simulink model "pfb_fft"  (Simulink 7.0)
settings: Solver=FixedStepDiscrete  SolverMode=SingleTasking  StartTime=0.0  StopTime=2500  RelTol=1e-3
libraries: xbsIndex_r4 x1144
(part 7 of 20)

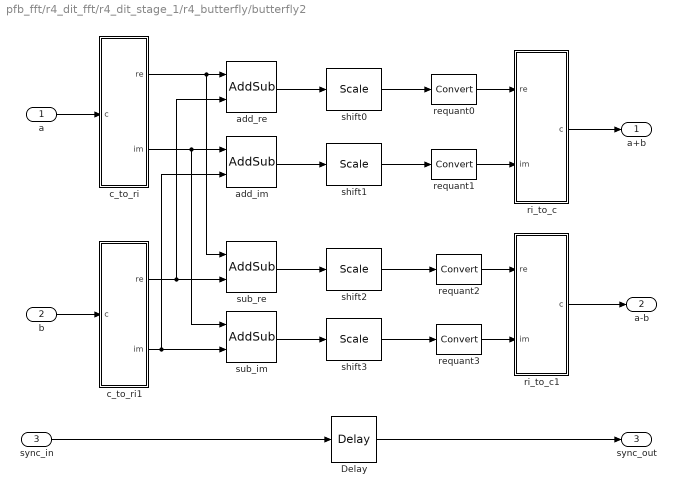
== system pfb_fft/r4_dit_fft/r4_dit_stage_1/r4_butterfly/butterfly2 ==
  a : Inport  OutDataType=sfix(16)  OutScaling=2^0
  b : Inport  Port=2  OutDataType=sfix(16)  OutScaling=2^0
  sync_in : Inport  Port=3  OutDataType=sfix(16)  OutScaling=2^0
  Delay : xbsIndex_r4/Delay  en=off  latency=1  dbl_ovrd=off  reg_retiming=off  block_type=delay
      settings: xl_area=[1 1 0 0 0 0 0]
  add_im : xbsIndex_r4/AddSub  mode=Addition  use_carryin=off  use_carryout=off  en=off  latency=1  precision=Full  arith_type=Unsigned  n_bits=8  bin_pt=2  quantization=Truncate  overflow=Wrap  dbl_ovrd=off  use_behavioral_HDL=on  pipelined=on  use_rpm=on  hw_selection=Fabric  block_type=addsub
      settings: xl_area=[6 11 0 11 0 0 0]  block_version=10.1.3
  add_re : xbsIndex_r4/AddSub  mode=Addition  use_carryin=off  use_carryout=off  en=off  latency=1  precision=Full  arith_type=Unsigned  n_bits=8  bin_pt=2  quantization=Truncate  overflow=Wrap  dbl_ovrd=off  use_behavioral_HDL=on  pipelined=on  use_rpm=on  hw_selection=Fabric  block_type=addsub
      settings: xl_area=[6 11 0 11 0 0 0]  block_version=10.1.3
  c_to_ri : Subsystem  mask(Complex to Real-Imag){n_bits=10, bin_pt=0}
      mask prompts: n_bits "Bit Width"; bin_pt "Binary Point"
      mask help: Outputs real and imaginary components of a complex input.
      settings: AttributesFormatString=10_0 r/i
      mask Help:
      | <pre>
      | Description::
      | 
      | Outputs real and imaginary components of a complex input.
      | Useful for simplifying interconnects.
      | See also: Real-Imag to Complex (ri_to_c)
      | 
      | Mask Parameters::
      | 
      | Bit Width (n_bits): Specifies the width of the real/imaginary components.
      | Assumed equal for both components.
      | 
      | Binary Point (bin_pt): Specifies the binary point location in the real/imaginary components.
      | Assumed equal for both components.
      | </pre>
  c_to_ri1 : Subsystem  mask(Complex to Real-Imag){n_bits=10, bin_pt=0}
      mask prompts: n_bits "Bit Width"; bin_pt "Binary Point"
      mask help: Outputs real and imaginary components of a complex input.
      settings: AttributesFormatString=10_0 r/i
      mask Help:
      | <pre>
      | Description::
      | 
      | Outputs real and imaginary components of a complex input.
      | Useful for simplifying interconnects.
      | See also: Real-Imag to Complex (ri_to_c)
      | 
      | Mask Parameters::
      | 
      | Bit Width (n_bits): Specifies the width of the real/imaginary components.
      | Assumed equal for both components.
      | 
      | Binary Point (bin_pt): Specifies the binary point location in the real/imaginary components.
      | Assumed equal for both components.
      | </pre>
  requant{0..3} (4 alike) : xbsIndex_r4/Convert  arith_type="Signed  (2's comp)"  n_bits=11  bin_pt=0  quantization=Truncate  overflow=Wrap  latency=0  dbl_ovrd=off  pipeline=on  block_type=convert
      settings: xl_area=[0 0 0 0 0 0 0]  block_version=10.1.3
  ri_to_c : Subsystem
      mask Type: Real-Imag to Complex
      mask Description: Concatenates real and imaginary inputs into a complex output.
      mask Help:
      | <pre>
      | Description::
      | 
      | Concatenates a real and imaginary input into a complex output.
      | Useful for simplifying interconnects.
      | See also: Complex to Real-Imag (c_to_ri)
      | 
      | Mask Parameters::
      | 
      | (N/A)
      | </pre>
  ri_to_c1 : Subsystem
      mask Type: Real-Imag to Complex
      mask Description: Concatenates real and imaginary inputs into a complex output.
      mask Help:
      | <pre>
      | Description::
      | 
      | Concatenates a real and imaginary input into a complex output.
      | Useful for simplifying interconnects.
      | See also: Complex to Real-Imag (c_to_ri)
      | 
      | Mask Parameters::
      | 
      | (N/A)
      | </pre>
  shift{0..3} (4 alike) : xbsIndex_r4/Scale  scale_factor=0  dbl_ovrd=off  block_type=scale
      settings: infoedit=Scales input by a power of two by adjusting the binary point position.<P><P>Hardware notes: In hardware this block costs nothing.  block_version=10.1.3
  sub_im : xbsIndex_r4/AddSub  mode=Subtraction  use_carryin=off  use_carryout=off  en=off  latency=1  precision=Full  arith_type=Unsigned  n_bits=8  bin_pt=2  quantization=Truncate  overflow=Wrap  dbl_ovrd=off  use_behavioral_HDL=on  pipelined=on  use_rpm=on  hw_selection=Fabric  block_type=addsub
      settings: xl_area=[6 11 0 11 0 0 0]  block_version=10.1.3
  sub_re : xbsIndex_r4/AddSub  mode=Subtraction  use_carryin=off  use_carryout=off  en=off  latency=1  precision=Full  arith_type=Unsigned  n_bits=8  bin_pt=2  quantization=Truncate  overflow=Wrap  dbl_ovrd=off  use_behavioral_HDL=on  pipelined=on  use_rpm=on  hw_selection=Fabric  block_type=addsub
      settings: xl_area=[6 11 0 11 0 0 0]  block_version=10.1.3
  a+b : Outport  OutDataType=sfix(16)  OutScaling=2^0
  a-b : Outport  Port=2  OutDataType=sfix(16)  OutScaling=2^0
  sync_out : Outport  Port=3  OutDataType=sfix(16)  OutScaling=2^0
  wires:
  shift3/1 -> requant3/1
  sub_im/1 -> shift3/1
  shift2/1 -> requant2/1
  sub_re/1 -> shift2/1
  shift1/1 -> requant1/1
  shift0/1 -> requant0/1
  requant3/1 -> ri_to_c1/2(im)
  requant2/1 -> ri_to_c1/1(re)
  requant1/1 -> ri_to_c/2(im)
  requant0/1 -> ri_to_c/1(re)
  Delay/1 -> sync_out/1
  sync_in/1 -> Delay/1
  ri_to_c1/1(c) -> a-b/1
  ri_to_c/1(c) -> a+b/1
  add_im/1 -> shift1/1
  add_re/1 -> shift0/1
  a/1 -> c_to_ri/1(c)
  c_to_ri/2(im) -> sub_im/1, add_im/1
  c_to_ri/1(re) -> sub_re/1, add_re/1
  c_to_ri1/2(im) -> add_im/2, sub_im/2
  c_to_ri1/1(re) -> add_re/2, sub_re/2
  b/1 -> c_to_ri1/1(c)

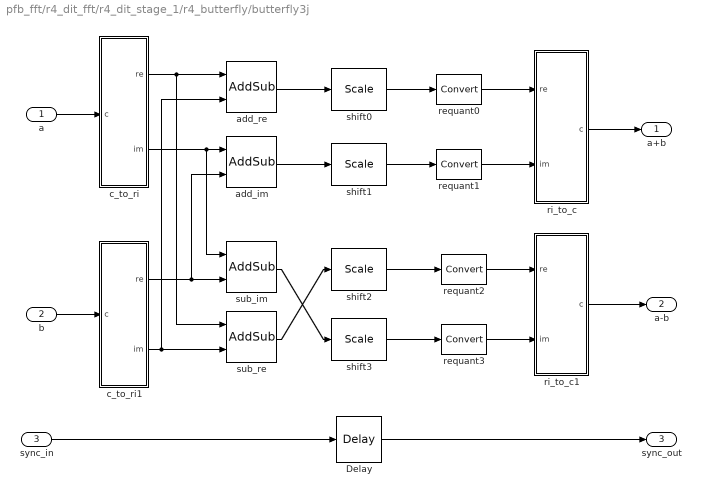
== system pfb_fft/r4_dit_fft/r4_dit_stage_1/r4_butterfly/butterfly3j ==
  a : Inport  OutDataType=sfix(16)  OutScaling=2^0
  b : Inport  Port=2  OutDataType=sfix(16)  OutScaling=2^0
  sync_in : Inport  Port=3  OutDataType=sfix(16)  OutScaling=2^0
  Delay : xbsIndex_r4/Delay  en=off  latency=1  dbl_ovrd=off  reg_retiming=off  block_type=delay
      settings: xl_area=[1 1 0 0 0 0 0]
  add_im : xbsIndex_r4/AddSub  mode=Subtraction  use_carryin=off  use_carryout=off  en=off  latency=1  precision=Full  arith_type=Unsigned  n_bits=8  bin_pt=2  quantization=Truncate  overflow=Wrap  dbl_ovrd=off  use_behavioral_HDL=on  pipelined=on  use_rpm=on  hw_selection=Fabric  block_type=addsub
      settings: xl_area=[6 11 0 11 0 0 0]  block_version=10.1.3
  add_re : xbsIndex_r4/AddSub  mode=Addition  use_carryin=off  use_carryout=off  en=off  latency=1  precision=Full  arith_type=Unsigned  n_bits=8  bin_pt=2  quantization=Truncate  overflow=Wrap  dbl_ovrd=off  use_behavioral_HDL=on  pipelined=on  use_rpm=on  hw_selection=Fabric  block_type=addsub
      settings: xl_area=[6 11 0 11 0 0 0]  block_version=10.1.3
  c_to_ri : Subsystem  mask(Complex to Real-Imag){n_bits=10, bin_pt=0}
      mask prompts: n_bits "Bit Width"; bin_pt "Binary Point"
      mask help: Outputs real and imaginary components of a complex input.
      settings: AttributesFormatString=10_0 r/i
      mask Help:
      | <pre>
      | Description::
      | 
      | Outputs real and imaginary components of a complex input.
      | Useful for simplifying interconnects.
      | See also: Real-Imag to Complex (ri_to_c)
      | 
      | Mask Parameters::
      | 
      | Bit Width (n_bits): Specifies the width of the real/imaginary components.
      | Assumed equal for both components.
      | 
      | Binary Point (bin_pt): Specifies the binary point location in the real/imaginary components.
      | Assumed equal for both components.
      | </pre>
  c_to_ri1 : Subsystem  mask(Complex to Real-Imag){n_bits=10, bin_pt=0}
      mask prompts: n_bits "Bit Width"; bin_pt "Binary Point"
      mask help: Outputs real and imaginary components of a complex input.
      settings: AttributesFormatString=10_0 r/i
      mask Help:
      | <pre>
      | Description::
      | 
      | Outputs real and imaginary components of a complex input.
      | Useful for simplifying interconnects.
      | See also: Real-Imag to Complex (ri_to_c)
      | 
      | Mask Parameters::
      | 
      | Bit Width (n_bits): Specifies the width of the real/imaginary components.
      | Assumed equal for both components.
      | 
      | Binary Point (bin_pt): Specifies the binary point location in the real/imaginary components.
      | Assumed equal for both components.
      | </pre>
  requant{0..3} (4 alike) : xbsIndex_r4/Convert  arith_type="Signed  (2's comp)"  n_bits=11  bin_pt=0  quantization=Truncate  overflow=Wrap  latency=0  dbl_ovrd=off  pipeline=on  block_type=convert
      settings: xl_area=[0 0 0 0 0 0 0]  block_version=10.1.3
  ri_to_c : Subsystem
      mask Type: Real-Imag to Complex
      mask Description: Concatenates real and imaginary inputs into a complex output.
      mask Help:
      | <pre>
      | Description::
      | 
      | Concatenates a real and imaginary input into a complex output.
      | Useful for simplifying interconnects.
      | See also: Complex to Real-Imag (c_to_ri)
      | 
      | Mask Parameters::
      | 
      | (N/A)
      | </pre>
  ri_to_c1 : Subsystem
      mask Type: Real-Imag to Complex
      mask Description: Concatenates real and imaginary inputs into a complex output.
      mask Help:
      | <pre>
      | Description::
      | 
      | Concatenates a real and imaginary input into a complex output.
      | Useful for simplifying interconnects.
      | See also: Complex to Real-Imag (c_to_ri)
      | 
      | Mask Parameters::
      | 
      | (N/A)
      | </pre>
  shift{0..3} (4 alike) : xbsIndex_r4/Scale  scale_factor=0  dbl_ovrd=off  block_type=scale
      settings: infoedit=Scales input by a power of two by adjusting the binary point position.<P><P>Hardware notes: In hardware this block costs nothing.  block_version=10.1.3
  sub_im : xbsIndex_r4/AddSub  mode=Addition  use_carryin=off  use_carryout=off  en=off  latency=1  precision=Full  arith_type=Unsigned  n_bits=8  bin_pt=2  quantization=Truncate  overflow=Wrap  dbl_ovrd=off  use_behavioral_HDL=on  pipelined=on  use_rpm=on  hw_selection=Fabric  block_type=addsub
      settings: xl_area=[6 11 0 11 0 0 0]  block_version=10.1.3
  sub_re : xbsIndex_r4/AddSub  mode=Subtraction  use_carryin=off  use_carryout=off  en=off  latency=1  precision=Full  arith_type=Unsigned  n_bits=8  bin_pt=2  quantization=Truncate  overflow=Wrap  dbl_ovrd=off  use_behavioral_HDL=on  pipelined=on  use_rpm=on  hw_selection=Fabric  block_type=addsub
      settings: xl_area=[6 11 0 11 0 0 0]  block_version=10.1.3
  a+b : Outport  OutDataType=sfix(16)  OutScaling=2^0
  a-b : Outport  Port=2  OutDataType=sfix(16)  OutScaling=2^0
  sync_out : Outport  Port=3  OutDataType=sfix(16)  OutScaling=2^0
  wires:
  requant3/1 -> ri_to_c1/2(im)
  requant2/1 -> ri_to_c1/1(re)
  requant1/1 -> ri_to_c/2(im)
  requant0/1 -> ri_to_c/1(re)
  shift3/1 -> requant3/1
  shift2/1 -> requant2/1
  shift1/1 -> requant1/1
  shift0/1 -> requant0/1
  sub_im/1 -> shift3/1
  sub_re/1 -> shift2/1
  b/1 -> c_to_ri1/1(c)
  c_to_ri1/1(re) -> add_im/2, sub_im/2
  c_to_ri1/2(im) -> add_re/2, sub_re/2
  c_to_ri/1(re) -> sub_re/1, add_re/1
  c_to_ri/2(im) -> sub_im/1, add_im/1
  a/1 -> c_to_ri/1(c)
  add_re/1 -> shift0/1
  add_im/1 -> shift1/1
  ri_to_c/1(c) -> a+b/1
  ri_to_c1/1(c) -> a-b/1
  sync_in/1 -> Delay/1
  Delay/1 -> sync_out/1

== system pfb_fft/r4_dit_fft/r4_dit_stage_2/quadplex_commutator/biplex_commutator_01 ==
  AloAhi : Inport  OutDataType=sfix(16)  OutScaling=2^0
  BloBhi : Inport  Port=2  OutDataType=sfix(16)  OutScaling=2^0
  sync_in : Inport  Port=3  OutDataType=sfix(16)  OutScaling=2^0
  Counter : xbsIndex_r4/Counter  cnt_type=Free Running  cnt_to=Inf  operation=Up  start_count=0  cnt_by_val=1  arith_type=Unsigned  n_bits=7  bin_pt=0  load_pin=off  rst=on  en=off  explicit_period=off  period=1  dbl_ovrd=off  use_behavioral_HDL=off  use_rpm=on  implementation=Fabric  block_type=counter
      settings: xl_area=[4 7 0 7 0 0 0]
  Delay : xbsIndex_r4/Delay  en=off  latency=65  dbl_ovrd=off  reg_retiming=off  block_type=delay
      settings: xl_area=[4 4 0 4 0 0 0]
  Mux : xbsIndex_r4/Mux  inputs=2  en=off  latency=1  precision=Full  arith_type="Signed  (2's comp)"  n_bits=8  bin_pt=2  quantization=Truncate  overflow=Wrap  dbl_ovrd=off  block_type=mux
      settings: xl_area=[11 22 0 22 0 0 0]
  Mux1 : xbsIndex_r4/Mux  inputs=2  en=off  latency=1  precision=Full  arith_type="Signed  (2's comp)"  n_bits=8  bin_pt=2  quantization=Truncate  overflow=Wrap  dbl_ovrd=off  block_type=mux
      settings: xl_area=[11 22 0 22 0 0 0]
  delay_b : Subsystem  mask(Complex Delay){delay_depth=64, n_bits=11, use_bram=on}
      mask prompts: delay_depth "Delay Depth"; n_bits "Bit Width"; use_bram "Use BRAM"
      mask help: A delay block that treats its input as complex, splits it into real and imaginary components, delays each component by a specified amount, and then re-joins them into a complex output. The underlying storage is user-selectable (either BRAM or SLR16 elements).
      settings: AttributesFormatString=|
      | depth = 64
      | delay bram
      mask Help:
      | <pre>
      | Description::
      | 
      | A delay block that treats its input as complex, splits it into real and imaginary components,
      | delays each component by a specified amount, and then re-joins them into a complex
      | output.  The underlying storage is user-selectable (either BRAM or SLR16 elements).
      | 
      | Mask Parameters::
      | 
      | Delay Depth (delay_depth): The length of the delay.
      | 
      | Bit Width (n_bits): Specifies the width of the real/imaginary components.
      | Width of each component is assumed equal.
      | 
      | Use BRAM (use_bram): Check this checkbox to implement the delay using BRAM.
      | If unchecked, the delay will be implemented using SLR16 elements.
      | </pre>
  delay_lo : Subsystem  mask(Complex Delay){delay_depth=64, n_bits=11, use_bram=on}
      mask prompts: delay_depth "Delay Depth"; n_bits "Bit Width"; use_bram "Use BRAM"
      mask help: A delay block that treats its input as complex, splits it into real and imaginary components, delays each component by a specified amount, and then re-joins them into a complex output. The underlying storage is user-selectable (either BRAM or SLR16 elements).
      settings: AttributesFormatString=|
      | depth = 64
      | delay bram
      mask Help:
      | <pre>
      | Description::
      | 
      | A delay block that treats its input as complex, splits it into real and imaginary components,
      | delays each component by a specified amount, and then re-joins them into a complex
      | output.  The underlying storage is user-selectable (either BRAM or SLR16 elements).
      | 
      | Mask Parameters::
      | 
      | Delay Depth (delay_depth): The length of the delay.
      | 
      | Bit Width (n_bits): Specifies the width of the real/imaginary components.
      | Width of each component is assumed equal.
      | 
      | Use BRAM (use_bram): Check this checkbox to implement the delay using BRAM.
      | If unchecked, the delay will be implemented using SLR16 elements.
      | </pre>
  top_bit : xbsIndex_r4/Slice  nbits=1  boolean_output=off  mode=Upper Bit Location + Width  bit1=0  base1=MSB of Input  bit0=0  base0=LSB of Input  dbl_ovrd=off  block_type=slice
      settings: infoedit="Extracts a given range of bits from each input sample and presents it at the output.  The output type is ordinarily unsigned with binary point at zero, but can be Boolean when the slice is one bit wide.<P><P>Hardware notes: In hardware this block costs nothing."  block_version=10.1.3
  AloBlo : Outport  OutDataType=sfix(16)  OutScaling=2^0
  AhiBhi : Outport  Port=2  OutDataType=sfix(16)  OutScaling=2^0
  sync_out : Outport  Port=3  OutDataType=sfix(16)  OutScaling=2^0
  wires:
  Delay/1 -> sync_out/1
  delay_lo/1(out) -> AloBlo/1
  Mux/1 -> delay_lo/1(in)
  delay_b/1(out) -> Mux/3, Mux1/2
  BloBhi/1 -> delay_b/1(in)
  Mux1/1 -> AhiBhi/1
  AloAhi/1 -> Mux1/3, Mux/2
  top_bit/1 -> Mux/1, Mux1/1
  Counter/1 -> top_bit/1
  sync_in/1 -> Delay/1, Counter/1

== system pfb_fft/r4_dit_fft/r4_dit_stage_2/quadplex_commutator/biplex_commutator_23 ==
  AloAhi : Inport  OutDataType=sfix(16)  OutScaling=2^0
  BloBhi : Inport  Port=2  OutDataType=sfix(16)  OutScaling=2^0
  sync_in : Inport  Port=3  OutDataType=sfix(16)  OutScaling=2^0
  Counter : xbsIndex_r4/Counter  cnt_type=Free Running  cnt_to=Inf  operation=Up  start_count=0  cnt_by_val=1  arith_type=Unsigned  n_bits=7  bin_pt=0  load_pin=off  rst=on  en=off  explicit_period=off  period=1  dbl_ovrd=off  use_behavioral_HDL=off  use_rpm=on  implementation=Fabric  block_type=counter
      settings: xl_area=[4 7 0 7 0 0 0]
  Delay : xbsIndex_r4/Delay  en=off  latency=65  dbl_ovrd=off  reg_retiming=off  block_type=delay
      settings: xl_area=[4 4 0 4 0 0 0]
  Mux : xbsIndex_r4/Mux  inputs=2  en=off  latency=1  precision=Full  arith_type="Signed  (2's comp)"  n_bits=8  bin_pt=2  quantization=Truncate  overflow=Wrap  dbl_ovrd=off  block_type=mux
      settings: xl_area=[11 22 0 22 0 0 0]
  Mux1 : xbsIndex_r4/Mux  inputs=2  en=off  latency=1  precision=Full  arith_type="Signed  (2's comp)"  n_bits=8  bin_pt=2  quantization=Truncate  overflow=Wrap  dbl_ovrd=off  block_type=mux
      settings: xl_area=[11 22 0 22 0 0 0]
  delay_b : Subsystem  mask(Complex Delay){delay_depth=64, n_bits=11, use_bram=on}
      mask prompts: delay_depth "Delay Depth"; n_bits "Bit Width"; use_bram "Use BRAM"
      mask help: A delay block that treats its input as complex, splits it into real and imaginary components, delays each component by a specified amount, and then re-joins them into a complex output. The underlying storage is user-selectable (either BRAM or SLR16 elements).
      settings: AttributesFormatString=|
      | depth = 64
      | delay bram
      mask Help:
      | <pre>
      | Description::
      | 
      | A delay block that treats its input as complex, splits it into real and imaginary components,
      | delays each component by a specified amount, and then re-joins them into a complex
      | output.  The underlying storage is user-selectable (either BRAM or SLR16 elements).
      | 
      | Mask Parameters::
      | 
      | Delay Depth (delay_depth): The length of the delay.
      | 
      | Bit Width (n_bits): Specifies the width of the real/imaginary components.
      | Width of each component is assumed equal.
      | 
      | Use BRAM (use_bram): Check this checkbox to implement the delay using BRAM.
      | If unchecked, the delay will be implemented using SLR16 elements.
      | </pre>
  delay_lo : Subsystem  mask(Complex Delay){delay_depth=64, n_bits=11, use_bram=on}
      mask prompts: delay_depth "Delay Depth"; n_bits "Bit Width"; use_bram "Use BRAM"
      mask help: A delay block that treats its input as complex, splits it into real and imaginary components, delays each component by a specified amount, and then re-joins them into a complex output. The underlying storage is user-selectable (either BRAM or SLR16 elements).
      settings: AttributesFormatString=|
      | depth = 64
      | delay bram
      mask Help:
      | <pre>
      | Description::
      | 
      | A delay block that treats its input as complex, splits it into real and imaginary components,
      | delays each component by a specified amount, and then re-joins them into a complex
      | output.  The underlying storage is user-selectable (either BRAM or SLR16 elements).
      | 
      | Mask Parameters::
      | 
      | Delay Depth (delay_depth): The length of the delay.
      | 
      | Bit Width (n_bits): Specifies the width of the real/imaginary components.
      | Width of each component is assumed equal.
      | 
      | Use BRAM (use_bram): Check this checkbox to implement the delay using BRAM.
      | If unchecked, the delay will be implemented using SLR16 elements.
      | </pre>
  top_bit : xbsIndex_r4/Slice  nbits=1  boolean_output=off  mode=Upper Bit Location + Width  bit1=0  base1=MSB of Input  bit0=0  base0=LSB of Input  dbl_ovrd=off  block_type=slice
      settings: infoedit="Extracts a given range of bits from each input sample and presents it at the output.  The output type is ordinarily unsigned with binary point at zero, but can be Boolean when the slice is one bit wide.<P><P>Hardware notes: In hardware this block costs nothing."  block_version=10.1.3
  AloBlo : Outport  OutDataType=sfix(16)  OutScaling=2^0
  AhiBhi : Outport  Port=2  OutDataType=sfix(16)  OutScaling=2^0
  sync_out : Outport  Port=3  OutDataType=sfix(16)  OutScaling=2^0
  wires:
  Delay/1 -> sync_out/1
  delay_lo/1(out) -> AloBlo/1
  Mux/1 -> delay_lo/1(in)
  delay_b/1(out) -> Mux/3, Mux1/2
  BloBhi/1 -> delay_b/1(in)
  Mux1/1 -> AhiBhi/1
  AloAhi/1 -> Mux1/3, Mux/2
  top_bit/1 -> Mux/1, Mux1/1
  Counter/1 -> top_bit/1
  sync_in/1 -> Delay/1, Counter/1

== system pfb_fft/r4_dit_fft/r4_dit_stage_2/quadplex_commutator/biplex_commutator_ac ==
  AloAhi : Inport  OutDataType=sfix(16)  OutScaling=2^0
  BloBhi : Inport  Port=2  OutDataType=sfix(16)  OutScaling=2^0
  sync_in : Inport  Port=3  OutDataType=sfix(16)  OutScaling=2^0
  Counter : xbsIndex_r4/Counter  cnt_type=Free Running  cnt_to=Inf  operation=Up  start_count=0  cnt_by_val=1  arith_type=Unsigned  n_bits=8  bin_pt=0  load_pin=off  rst=on  en=off  explicit_period=off  period=1  dbl_ovrd=off  use_behavioral_HDL=off  use_rpm=on  implementation=Fabric  block_type=counter
      settings: xl_area=[4 8 0 8 0 0 0]
  Delay : xbsIndex_r4/Delay  en=off  latency=129  dbl_ovrd=off  reg_retiming=off  block_type=delay
      settings: xl_area=[8 8 0 8 0 0 0]
  Mux : xbsIndex_r4/Mux  inputs=2  en=off  latency=1  precision=Full  arith_type="Signed  (2's comp)"  n_bits=8  bin_pt=2  quantization=Truncate  overflow=Wrap  dbl_ovrd=off  block_type=mux
      settings: xl_area=[11 22 0 22 0 0 0]
  Mux1 : xbsIndex_r4/Mux  inputs=2  en=off  latency=1  precision=Full  arith_type="Signed  (2's comp)"  n_bits=8  bin_pt=2  quantization=Truncate  overflow=Wrap  dbl_ovrd=off  block_type=mux
      settings: xl_area=[11 22 0 22 0 0 0]
  delay_b : Subsystem  mask(Complex Delay){delay_depth=128, n_bits=11, use_bram=on}
      mask prompts: delay_depth "Delay Depth"; n_bits "Bit Width"; use_bram "Use BRAM"
      mask help: A delay block that treats its input as complex, splits it into real and imaginary components, delays each component by a specified amount, and then re-joins them into a complex output. The underlying storage is user-selectable (either BRAM or SLR16 elements).
      settings: AttributesFormatString=|
      | depth = 128
      | delay bram
      mask Help:
      | <pre>
      | Description::
      | 
      | A delay block that treats its input as complex, splits it into real and imaginary components,
      | delays each component by a specified amount, and then re-joins them into a complex
      | output.  The underlying storage is user-selectable (either BRAM or SLR16 elements).
      | 
      | Mask Parameters::
      | 
      | Delay Depth (delay_depth): The length of the delay.
      | 
      | Bit Width (n_bits): Specifies the width of the real/imaginary components.
      | Width of each component is assumed equal.
      | 
      | Use BRAM (use_bram): Check this checkbox to implement the delay using BRAM.
      | If unchecked, the delay will be implemented using SLR16 elements.
      | </pre>
  delay_lo : Subsystem  mask(Complex Delay){delay_depth=128, n_bits=11, use_bram=on}
      mask prompts: delay_depth "Delay Depth"; n_bits "Bit Width"; use_bram "Use BRAM"
      mask help: A delay block that treats its input as complex, splits it into real and imaginary components, delays each component by a specified amount, and then re-joins them into a complex output. The underlying storage is user-selectable (either BRAM or SLR16 elements).
      settings: AttributesFormatString=|
      | depth = 128
      | delay bram
      mask Help:
      | <pre>
      | Description::
      | 
      | A delay block that treats its input as complex, splits it into real and imaginary components,
      | delays each component by a specified amount, and then re-joins them into a complex
      | output.  The underlying storage is user-selectable (either BRAM or SLR16 elements).
      | 
      | Mask Parameters::
      | 
      | Delay Depth (delay_depth): The length of the delay.
      | 
      | Bit Width (n_bits): Specifies the width of the real/imaginary components.
      | Width of each component is assumed equal.
      | 
      | Use BRAM (use_bram): Check this checkbox to implement the delay using BRAM.
      | If unchecked, the delay will be implemented using SLR16 elements.
      | </pre>
  top_bit : xbsIndex_r4/Slice  nbits=1  boolean_output=off  mode=Upper Bit Location + Width  bit1=0  base1=MSB of Input  bit0=0  base0=LSB of Input  dbl_ovrd=off  block_type=slice
      settings: infoedit="Extracts a given range of bits from each input sample and presents it at the output.  The output type is ordinarily unsigned with binary point at zero, but can be Boolean when the slice is one bit wide.<P><P>Hardware notes: In hardware this block costs nothing."  block_version=10.1.3
  AloBlo : Outport  OutDataType=sfix(16)  OutScaling=2^0
  AhiBhi : Outport  Port=2  OutDataType=sfix(16)  OutScaling=2^0
  sync_out : Outport  Port=3  OutDataType=sfix(16)  OutScaling=2^0
  wires:
  Delay/1 -> sync_out/1
  delay_lo/1(out) -> AloBlo/1
  Mux/1 -> delay_lo/1(in)
  delay_b/1(out) -> Mux/3, Mux1/2
  BloBhi/1 -> delay_b/1(in)
  Mux1/1 -> AhiBhi/1
  AloAhi/1 -> Mux1/3, Mux/2
  top_bit/1 -> Mux/1, Mux1/1
  Counter/1 -> top_bit/1
  sync_in/1 -> Delay/1, Counter/1

== system pfb_fft/r4_dit_fft/r4_dit_stage_2/quadplex_commutator/biplex_commutator_bd ==
  AloAhi : Inport  OutDataType=sfix(16)  OutScaling=2^0
  BloBhi : Inport  Port=2  OutDataType=sfix(16)  OutScaling=2^0
  sync_in : Inport  Port=3  OutDataType=sfix(16)  OutScaling=2^0
  Counter : xbsIndex_r4/Counter  cnt_type=Free Running  cnt_to=Inf  operation=Up  start_count=0  cnt_by_val=1  arith_type=Unsigned  n_bits=8  bin_pt=0  load_pin=off  rst=on  en=off  explicit_period=off  period=1  dbl_ovrd=off  use_behavioral_HDL=off  use_rpm=on  implementation=Fabric  block_type=counter
      settings: xl_area=[4 8 0 8 0 0 0]
  Delay : xbsIndex_r4/Delay  en=off  latency=129  dbl_ovrd=off  reg_retiming=off  block_type=delay
      settings: xl_area=[8 8 0 8 0 0 0]
  Mux : xbsIndex_r4/Mux  inputs=2  en=off  latency=1  precision=Full  arith_type="Signed  (2's comp)"  n_bits=8  bin_pt=2  quantization=Truncate  overflow=Wrap  dbl_ovrd=off  block_type=mux
      settings: xl_area=[11 22 0 22 0 0 0]
  Mux1 : xbsIndex_r4/Mux  inputs=2  en=off  latency=1  precision=Full  arith_type="Signed  (2's comp)"  n_bits=8  bin_pt=2  quantization=Truncate  overflow=Wrap  dbl_ovrd=off  block_type=mux
      settings: xl_area=[11 22 0 22 0 0 0]
  delay_b : Subsystem  mask(Complex Delay){delay_depth=128, n_bits=11, use_bram=on}
      mask prompts: delay_depth "Delay Depth"; n_bits "Bit Width"; use_bram "Use BRAM"
      mask help: A delay block that treats its input as complex, splits it into real and imaginary components, delays each component by a specified amount, and then re-joins them into a complex output. The underlying storage is user-selectable (either BRAM or SLR16 elements).
      settings: AttributesFormatString=|
      | depth = 128
      | delay bram
      mask Help:
      | <pre>
      | Description::
      | 
      | A delay block that treats its input as complex, splits it into real and imaginary components,
      | delays each component by a specified amount, and then re-joins them into a complex
      | output.  The underlying storage is user-selectable (either BRAM or SLR16 elements).
      | 
      | Mask Parameters::
      | 
      | Delay Depth (delay_depth): The length of the delay.
      | 
      | Bit Width (n_bits): Specifies the width of the real/imaginary components.
      | Width of each component is assumed equal.
      | 
      | Use BRAM (use_bram): Check this checkbox to implement the delay using BRAM.
      | If unchecked, the delay will be implemented using SLR16 elements.
      | </pre>
  delay_lo : Subsystem  mask(Complex Delay){delay_depth=128, n_bits=11, use_bram=on}
      mask prompts: delay_depth "Delay Depth"; n_bits "Bit Width"; use_bram "Use BRAM"
      mask help: A delay block that treats its input as complex, splits it into real and imaginary components, delays each component by a specified amount, and then re-joins them into a complex output. The underlying storage is user-selectable (either BRAM or SLR16 elements).
      settings: AttributesFormatString=|
      | depth = 128
      | delay bram
      mask Help:
      | <pre>
      | Description::
      | 
      | A delay block that treats its input as complex, splits it into real and imaginary components,
      | delays each component by a specified amount, and then re-joins them into a complex
      | output.  The underlying storage is user-selectable (either BRAM or SLR16 elements).
      | 
      | Mask Parameters::
      | 
      | Delay Depth (delay_depth): The length of the delay.
      | 
      | Bit Width (n_bits): Specifies the width of the real/imaginary components.
      | Width of each component is assumed equal.
      | 
      | Use BRAM (use_bram): Check this checkbox to implement the delay using BRAM.
      | If unchecked, the delay will be implemented using SLR16 elements.
      | </pre>
  top_bit : xbsIndex_r4/Slice  nbits=1  boolean_output=off  mode=Upper Bit Location + Width  bit1=0  base1=MSB of Input  bit0=0  base0=LSB of Input  dbl_ovrd=off  block_type=slice
      settings: infoedit="Extracts a given range of bits from each input sample and presents it at the output.  The output type is ordinarily unsigned with binary point at zero, but can be Boolean when the slice is one bit wide.<P><P>Hardware notes: In hardware this block costs nothing."  block_version=10.1.3
  AloBlo : Outport  OutDataType=sfix(16)  OutScaling=2^0
  AhiBhi : Outport  Port=2  OutDataType=sfix(16)  OutScaling=2^0
  sync_out : Outport  Port=3  OutDataType=sfix(16)  OutScaling=2^0
  wires:
  Delay/1 -> sync_out/1
  delay_lo/1(out) -> AloBlo/1
  Mux/1 -> delay_lo/1(in)
  delay_b/1(out) -> Mux/3, Mux1/2
  BloBhi/1 -> delay_b/1(in)
  Mux1/1 -> AhiBhi/1
  AloAhi/1 -> Mux1/3, Mux/2
  top_bit/1 -> Mux/1, Mux1/1
  Counter/1 -> top_bit/1
  sync_in/1 -> Delay/1, Counter/1

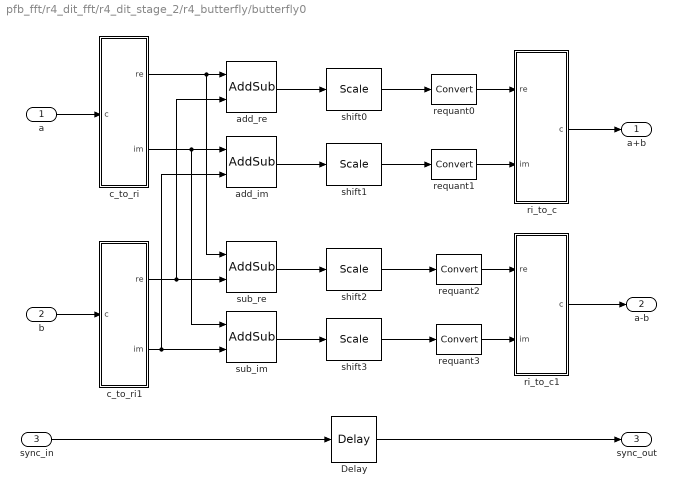
== system pfb_fft/r4_dit_fft/r4_dit_stage_2/r4_butterfly/butterfly0 ==
  a : Inport  OutDataType=sfix(16)  OutScaling=2^0
  b : Inport  Port=2  OutDataType=sfix(16)  OutScaling=2^0
  sync_in : Inport  Port=3  OutDataType=sfix(16)  OutScaling=2^0
  Delay : xbsIndex_r4/Delay  en=off  latency=1  dbl_ovrd=off  reg_retiming=off  block_type=delay
      settings: xl_area=[1 1 0 0 0 0 0]
  add_im : xbsIndex_r4/AddSub  mode=Addition  use_carryin=off  use_carryout=off  en=off  latency=1  precision=Full  arith_type=Unsigned  n_bits=8  bin_pt=2  quantization=Truncate  overflow=Wrap  dbl_ovrd=off  use_behavioral_HDL=on  pipelined=on  use_rpm=on  hw_selection=Fabric  block_type=addsub
      settings: xl_area=[6 12 0 12 0 0 0]  block_version=10.1.3
  add_re : xbsIndex_r4/AddSub  mode=Addition  use_carryin=off  use_carryout=off  en=off  latency=1  precision=Full  arith_type=Unsigned  n_bits=8  bin_pt=2  quantization=Truncate  overflow=Wrap  dbl_ovrd=off  use_behavioral_HDL=on  pipelined=on  use_rpm=on  hw_selection=Fabric  block_type=addsub
      settings: xl_area=[6 12 0 12 0 0 0]  block_version=10.1.3
  c_to_ri : Subsystem  mask(Complex to Real-Imag){n_bits=11, bin_pt=0}
      mask prompts: n_bits "Bit Width"; bin_pt "Binary Point"
      mask help: Outputs real and imaginary components of a complex input.
      settings: AttributesFormatString=11_0 r/i
      mask Help:
      | <pre>
      | Description::
      | 
      | Outputs real and imaginary components of a complex input.
      | Useful for simplifying interconnects.
      | See also: Real-Imag to Complex (ri_to_c)
      | 
      | Mask Parameters::
      | 
      | Bit Width (n_bits): Specifies the width of the real/imaginary components.
      | Assumed equal for both components.
      | 
      | Binary Point (bin_pt): Specifies the binary point location in the real/imaginary components.
      | Assumed equal for both components.
      | </pre>
  c_to_ri1 : Subsystem  mask(Complex to Real-Imag){n_bits=11, bin_pt=0}
      mask prompts: n_bits "Bit Width"; bin_pt "Binary Point"
      mask help: Outputs real and imaginary components of a complex input.
      settings: AttributesFormatString=11_0 r/i
      mask Help:
      | <pre>
      | Description::
      | 
      | Outputs real and imaginary components of a complex input.
      | Useful for simplifying interconnects.
      | See also: Real-Imag to Complex (ri_to_c)
      | 
      | Mask Parameters::
      | 
      | Bit Width (n_bits): Specifies the width of the real/imaginary components.
      | Assumed equal for both components.
      | 
      | Binary Point (bin_pt): Specifies the binary point location in the real/imaginary components.
      | Assumed equal for both components.
      | </pre>
  requant{0..3} (4 alike) : xbsIndex_r4/Convert  arith_type="Signed  (2's comp)"  n_bits=12  bin_pt=0  quantization=Truncate  overflow=Wrap  latency=0  dbl_ovrd=off  pipeline=on  block_type=convert
      settings: xl_area=[0 0 0 0 0 0 0]  block_version=10.1.3
  ri_to_c : Subsystem
      mask Type: Real-Imag to Complex
      mask Description: Concatenates real and imaginary inputs into a complex output.
      mask Help:
      | <pre>
      | Description::
      | 
      | Concatenates a real and imaginary input into a complex output.
      | Useful for simplifying interconnects.
      | See also: Complex to Real-Imag (c_to_ri)
      | 
      | Mask Parameters::
      | 
      | (N/A)
      | </pre>
  ri_to_c1 : Subsystem
      mask Type: Real-Imag to Complex
      mask Description: Concatenates real and imaginary inputs into a complex output.
      mask Help:
      | <pre>
      | Description::
      | 
      | Concatenates a real and imaginary input into a complex output.
      | Useful for simplifying interconnects.
      | See also: Complex to Real-Imag (c_to_ri)
      | 
      | Mask Parameters::
      | 
      | (N/A)
      | </pre>
  shift{0..3} (4 alike) : xbsIndex_r4/Scale  scale_factor=0  dbl_ovrd=off  block_type=scale
      settings: infoedit=Scales input by a power of two by adjusting the binary point position.<P><P>Hardware notes: In hardware this block costs nothing.  block_version=10.1.3
  sub_im : xbsIndex_r4/AddSub  mode=Subtraction  use_carryin=off  use_carryout=off  en=off  latency=1  precision=Full  arith_type=Unsigned  n_bits=8  bin_pt=2  quantization=Truncate  overflow=Wrap  dbl_ovrd=off  use_behavioral_HDL=on  pipelined=on  use_rpm=on  hw_selection=Fabric  block_type=addsub
      settings: xl_area=[6 12 0 12 0 0 0]  block_version=10.1.3
  sub_re : xbsIndex_r4/AddSub  mode=Subtraction  use_carryin=off  use_carryout=off  en=off  latency=1  precision=Full  arith_type=Unsigned  n_bits=8  bin_pt=2  quantization=Truncate  overflow=Wrap  dbl_ovrd=off  use_behavioral_HDL=on  pipelined=on  use_rpm=on  hw_selection=Fabric  block_type=addsub
      settings: xl_area=[6 12 0 12 0 0 0]  block_version=10.1.3
  a+b : Outport  OutDataType=sfix(16)  OutScaling=2^0
  a-b : Outport  Port=2  OutDataType=sfix(16)  OutScaling=2^0
  sync_out : Outport  Port=3  OutDataType=sfix(16)  OutScaling=2^0
  wires:
  shift3/1 -> requant3/1
  sub_im/1 -> shift3/1
  shift2/1 -> requant2/1
  sub_re/1 -> shift2/1
  shift1/1 -> requant1/1
  shift0/1 -> requant0/1
  requant3/1 -> ri_to_c1/2(im)
  requant2/1 -> ri_to_c1/1(re)
  requant1/1 -> ri_to_c/2(im)
  requant0/1 -> ri_to_c/1(re)
  Delay/1 -> sync_out/1
  sync_in/1 -> Delay/1
  ri_to_c1/1(c) -> a-b/1
  ri_to_c/1(c) -> a+b/1
  add_im/1 -> shift1/1
  add_re/1 -> shift0/1
  a/1 -> c_to_ri/1(c)
  c_to_ri/2(im) -> sub_im/1, add_im/1
  c_to_ri/1(re) -> sub_re/1, add_re/1
  c_to_ri1/2(im) -> add_im/2, sub_im/2
  c_to_ri1/1(re) -> add_re/2, sub_re/2
  b/1 -> c_to_ri1/1(c)

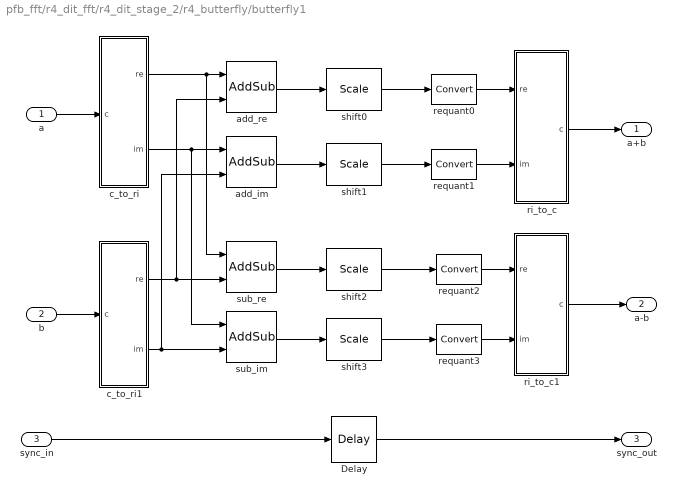
== system pfb_fft/r4_dit_fft/r4_dit_stage_2/r4_butterfly/butterfly1 ==
  a : Inport  OutDataType=sfix(16)  OutScaling=2^0
  b : Inport  Port=2  OutDataType=sfix(16)  OutScaling=2^0
  sync_in : Inport  Port=3  OutDataType=sfix(16)  OutScaling=2^0
  Delay : xbsIndex_r4/Delay  en=off  latency=1  dbl_ovrd=off  reg_retiming=off  block_type=delay
      settings: xl_area=[1 1 0 0 0 0 0]
  add_im : xbsIndex_r4/AddSub  mode=Addition  use_carryin=off  use_carryout=off  en=off  latency=1  precision=Full  arith_type=Unsigned  n_bits=8  bin_pt=2  quantization=Truncate  overflow=Wrap  dbl_ovrd=off  use_behavioral_HDL=on  pipelined=on  use_rpm=on  hw_selection=Fabric  block_type=addsub
      settings: xl_area=[6 12 0 12 0 0 0]  block_version=10.1.3
  add_re : xbsIndex_r4/AddSub  mode=Addition  use_carryin=off  use_carryout=off  en=off  latency=1  precision=Full  arith_type=Unsigned  n_bits=8  bin_pt=2  quantization=Truncate  overflow=Wrap  dbl_ovrd=off  use_behavioral_HDL=on  pipelined=on  use_rpm=on  hw_selection=Fabric  block_type=addsub
      settings: xl_area=[6 12 0 12 0 0 0]  block_version=10.1.3
  c_to_ri : Subsystem  mask(Complex to Real-Imag){n_bits=11, bin_pt=0}
      mask prompts: n_bits "Bit Width"; bin_pt "Binary Point"
      mask help: Outputs real and imaginary components of a complex input.
      settings: AttributesFormatString=11_0 r/i
      mask Help:
      | <pre>
      | Description::
      | 
      | Outputs real and imaginary components of a complex input.
      | Useful for simplifying interconnects.
      | See also: Real-Imag to Complex (ri_to_c)
      | 
      | Mask Parameters::
      | 
      | Bit Width (n_bits): Specifies the width of the real/imaginary components.
      | Assumed equal for both components.
      | 
      | Binary Point (bin_pt): Specifies the binary point location in the real/imaginary components.
      | Assumed equal for both components.
      | </pre>
  c_to_ri1 : Subsystem  mask(Complex to Real-Imag){n_bits=11, bin_pt=0}
      mask prompts: n_bits "Bit Width"; bin_pt "Binary Point"
      mask help: Outputs real and imaginary components of a complex input.
      settings: AttributesFormatString=11_0 r/i
      mask Help:
      | <pre>
      | Description::
      | 
      | Outputs real and imaginary components of a complex input.
      | Useful for simplifying interconnects.
      | See also: Real-Imag to Complex (ri_to_c)
      | 
      | Mask Parameters::
      | 
      | Bit Width (n_bits): Specifies the width of the real/imaginary components.
      | Assumed equal for both components.
      | 
      | Binary Point (bin_pt): Specifies the binary point location in the real/imaginary components.
      | Assumed equal for both components.
      | </pre>
  requant{0..3} (4 alike) : xbsIndex_r4/Convert  arith_type="Signed  (2's comp)"  n_bits=12  bin_pt=0  quantization=Truncate  overflow=Wrap  latency=0  dbl_ovrd=off  pipeline=on  block_type=convert
      settings: xl_area=[0 0 0 0 0 0 0]  block_version=10.1.3
  ri_to_c : Subsystem
      mask Type: Real-Imag to Complex
      mask Description: Concatenates real and imaginary inputs into a complex output.
      mask Help:
      | <pre>
      | Description::
      | 
      | Concatenates a real and imaginary input into a complex output.
      | Useful for simplifying interconnects.
      | See also: Complex to Real-Imag (c_to_ri)
      | 
      | Mask Parameters::
      | 
      | (N/A)
      | </pre>
  ri_to_c1 : Subsystem
      mask Type: Real-Imag to Complex
      mask Description: Concatenates real and imaginary inputs into a complex output.
      mask Help:
      | <pre>
      | Description::
      | 
      | Concatenates a real and imaginary input into a complex output.
      | Useful for simplifying interconnects.
      | See also: Complex to Real-Imag (c_to_ri)
      | 
      | Mask Parameters::
      | 
      | (N/A)
      | </pre>
  shift{0..3} (4 alike) : xbsIndex_r4/Scale  scale_factor=0  dbl_ovrd=off  block_type=scale
      settings: infoedit=Scales input by a power of two by adjusting the binary point position.<P><P>Hardware notes: In hardware this block costs nothing.  block_version=10.1.3
  sub_im : xbsIndex_r4/AddSub  mode=Subtraction  use_carryin=off  use_carryout=off  en=off  latency=1  precision=Full  arith_type=Unsigned  n_bits=8  bin_pt=2  quantization=Truncate  overflow=Wrap  dbl_ovrd=off  use_behavioral_HDL=on  pipelined=on  use_rpm=on  hw_selection=Fabric  block_type=addsub
      settings: xl_area=[6 12 0 12 0 0 0]  block_version=10.1.3
  sub_re : xbsIndex_r4/AddSub  mode=Subtraction  use_carryin=off  use_carryout=off  en=off  latency=1  precision=Full  arith_type=Unsigned  n_bits=8  bin_pt=2  quantization=Truncate  overflow=Wrap  dbl_ovrd=off  use_behavioral_HDL=on  pipelined=on  use_rpm=on  hw_selection=Fabric  block_type=addsub
      settings: xl_area=[6 12 0 12 0 0 0]  block_version=10.1.3
  a+b : Outport  OutDataType=sfix(16)  OutScaling=2^0
  a-b : Outport  Port=2  OutDataType=sfix(16)  OutScaling=2^0
  sync_out : Outport  Port=3  OutDataType=sfix(16)  OutScaling=2^0
  wires:
  shift3/1 -> requant3/1
  sub_im/1 -> shift3/1
  shift2/1 -> requant2/1
  sub_re/1 -> shift2/1
  shift1/1 -> requant1/1
  shift0/1 -> requant0/1
  requant3/1 -> ri_to_c1/2(im)
  requant2/1 -> ri_to_c1/1(re)
  requant1/1 -> ri_to_c/2(im)
  requant0/1 -> ri_to_c/1(re)
  Delay/1 -> sync_out/1
  sync_in/1 -> Delay/1
  ri_to_c1/1(c) -> a-b/1
  ri_to_c/1(c) -> a+b/1
  add_im/1 -> shift1/1
  add_re/1 -> shift0/1
  a/1 -> c_to_ri/1(c)
  c_to_ri/2(im) -> sub_im/1, add_im/1
  c_to_ri/1(re) -> sub_re/1, add_re/1
  c_to_ri1/2(im) -> add_im/2, sub_im/2
  c_to_ri1/1(re) -> add_re/2, sub_re/2
  b/1 -> c_to_ri1/1(c)

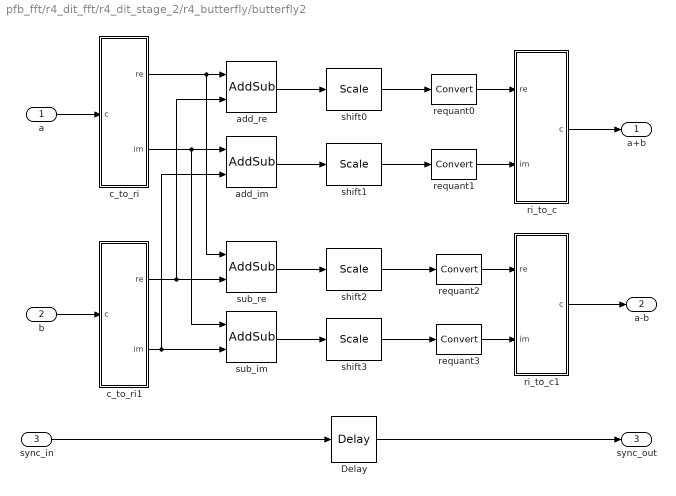
== system pfb_fft/r4_dit_fft/r4_dit_stage_2/r4_butterfly/butterfly2 ==
  a : Inport  OutDataType=sfix(16)  OutScaling=2^0
  b : Inport  Port=2  OutDataType=sfix(16)  OutScaling=2^0
  sync_in : Inport  Port=3  OutDataType=sfix(16)  OutScaling=2^0
  Delay : xbsIndex_r4/Delay  en=off  latency=1  dbl_ovrd=off  reg_retiming=off  block_type=delay
      settings: xl_area=[1 1 0 0 0 0 0]
  add_im : xbsIndex_r4/AddSub  mode=Addition  use_carryin=off  use_carryout=off  en=off  latency=1  precision=Full  arith_type=Unsigned  n_bits=8  bin_pt=2  quantization=Truncate  overflow=Wrap  dbl_ovrd=off  use_behavioral_HDL=on  pipelined=on  use_rpm=on  hw_selection=Fabric  block_type=addsub
      settings: xl_area=[7 13 0 13 0 0 0]  block_version=10.1.3
  add_re : xbsIndex_r4/AddSub  mode=Addition  use_carryin=off  use_carryout=off  en=off  latency=1  precision=Full  arith_type=Unsigned  n_bits=8  bin_pt=2  quantization=Truncate  overflow=Wrap  dbl_ovrd=off  use_behavioral_HDL=on  pipelined=on  use_rpm=on  hw_selection=Fabric  block_type=addsub
      settings: xl_area=[7 13 0 13 0 0 0]  block_version=10.1.3
  c_to_ri : Subsystem  mask(Complex to Real-Imag){n_bits=12, bin_pt=0}
      mask prompts: n_bits "Bit Width"; bin_pt "Binary Point"
      mask help: Outputs real and imaginary components of a complex input.
      settings: AttributesFormatString=12_0 r/i
      mask Help:
      | <pre>
      | Description::
      | 
      | Outputs real and imaginary components of a complex input.
      | Useful for simplifying interconnects.
      | See also: Real-Imag to Complex (ri_to_c)
      | 
      | Mask Parameters::
      | 
      | Bit Width (n_bits): Specifies the width of the real/imaginary components.
      | Assumed equal for both components.
      | 
      | Binary Point (bin_pt): Specifies the binary point location in the real/imaginary components.
      | Assumed equal for both components.
      | </pre>
  c_to_ri1 : Subsystem  mask(Complex to Real-Imag){n_bits=12, bin_pt=0}
      mask prompts: n_bits "Bit Width"; bin_pt "Binary Point"
      mask help: Outputs real and imaginary components of a complex input.
      settings: AttributesFormatString=12_0 r/i
      mask Help:
      | <pre>
      | Description::
      | 
      | Outputs real and imaginary components of a complex input.
      | Useful for simplifying interconnects.
      | See also: Real-Imag to Complex (ri_to_c)
      | 
      | Mask Parameters::
      | 
      | Bit Width (n_bits): Specifies the width of the real/imaginary components.
      | Assumed equal for both components.
      | 
      | Binary Point (bin_pt): Specifies the binary point location in the real/imaginary components.
      | Assumed equal for both components.
      | </pre>
  requant{0..3} (4 alike) : xbsIndex_r4/Convert  arith_type="Signed  (2's comp)"  n_bits=13  bin_pt=0  quantization=Truncate  overflow=Wrap  latency=0  dbl_ovrd=off  pipeline=on  block_type=convert
      settings: xl_area=[0 0 0 0 0 0 0]  block_version=10.1.3
  ri_to_c : Subsystem
      mask Type: Real-Imag to Complex
      mask Description: Concatenates real and imaginary inputs into a complex output.
      mask Help:
      | <pre>
      | Description::
      | 
      | Concatenates a real and imaginary input into a complex output.
      | Useful for simplifying interconnects.
      | See also: Complex to Real-Imag (c_to_ri)
      | 
      | Mask Parameters::
      | 
      | (N/A)
      | </pre>
  ri_to_c1 : Subsystem
      mask Type: Real-Imag to Complex
      mask Description: Concatenates real and imaginary inputs into a complex output.
      mask Help:
      | <pre>
      | Description::
      | 
      | Concatenates a real and imaginary input into a complex output.
      | Useful for simplifying interconnects.
      | See also: Complex to Real-Imag (c_to_ri)
      | 
      | Mask Parameters::
      | 
      | (N/A)
      | </pre>
  shift{0..3} (4 alike) : xbsIndex_r4/Scale  scale_factor=0  dbl_ovrd=off  block_type=scale
      settings: infoedit=Scales input by a power of two by adjusting the binary point position.<P><P>Hardware notes: In hardware this block costs nothing.  block_version=10.1.3
  sub_im : xbsIndex_r4/AddSub  mode=Subtraction  use_carryin=off  use_carryout=off  en=off  latency=1  precision=Full  arith_type=Unsigned  n_bits=8  bin_pt=2  quantization=Truncate  overflow=Wrap  dbl_ovrd=off  use_behavioral_HDL=on  pipelined=on  use_rpm=on  hw_selection=Fabric  block_type=addsub
      settings: xl_area=[7 13 0 13 0 0 0]  block_version=10.1.3
  sub_re : xbsIndex_r4/AddSub  mode=Subtraction  use_carryin=off  use_carryout=off  en=off  latency=1  precision=Full  arith_type=Unsigned  n_bits=8  bin_pt=2  quantization=Truncate  overflow=Wrap  dbl_ovrd=off  use_behavioral_HDL=on  pipelined=on  use_rpm=on  hw_selection=Fabric  block_type=addsub
      settings: xl_area=[7 13 0 13 0 0 0]  block_version=10.1.3
  a+b : Outport  OutDataType=sfix(16)  OutScaling=2^0
  a-b : Outport  Port=2  OutDataType=sfix(16)  OutScaling=2^0
  sync_out : Outport  Port=3  OutDataType=sfix(16)  OutScaling=2^0
  wires:
  shift3/1 -> requant3/1
  sub_im/1 -> shift3/1
  shift2/1 -> requant2/1
  sub_re/1 -> shift2/1
  shift1/1 -> requant1/1
  shift0/1 -> requant0/1
  requant3/1 -> ri_to_c1/2(im)
  requant2/1 -> ri_to_c1/1(re)
  requant1/1 -> ri_to_c/2(im)
  requant0/1 -> ri_to_c/1(re)
  Delay/1 -> sync_out/1
  sync_in/1 -> Delay/1
  ri_to_c1/1(c) -> a-b/1
  ri_to_c/1(c) -> a+b/1
  add_im/1 -> shift1/1
  add_re/1 -> shift0/1
  a/1 -> c_to_ri/1(c)
  c_to_ri/2(im) -> sub_im/1, add_im/1
  c_to_ri/1(re) -> sub_re/1, add_re/1
  c_to_ri1/2(im) -> add_im/2, sub_im/2
  c_to_ri1/1(re) -> add_re/2, sub_re/2
  b/1 -> c_to_ri1/1(c)
